simulink model "FilterTest3"  (R2013a)
settings: Solver=FixedStepDiscrete  StartTime=0.0  StopTime=30  RelTol=1e-3
values from neighbouring files (symbols this model uses):
  Ts = 1/100    (= 0.01)    [DataAnalysis.m]
undefined symbols (not defined in the file): a1_1, a1_2, a2_1, a2_2, b0_1, b0_2, b1_1, b1_2, b2_1, b2_2, N, p0_1, p0_2
settings Model: Creator=jban039  LastModifiedBy=jban039

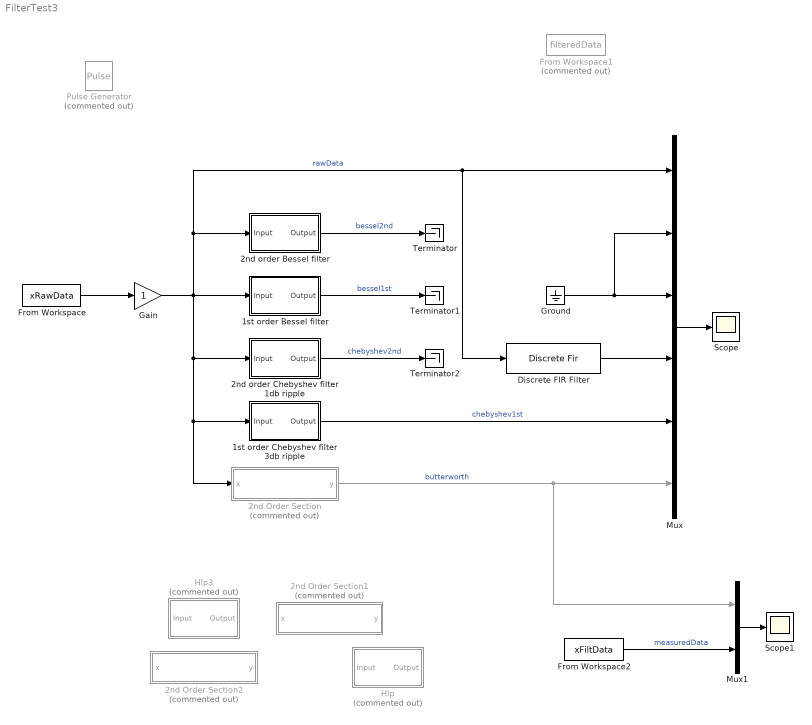
== system FilterTest3 ==
  1st order Bessel filter : Subsystem  Tag=FilterWizardSubSystem
      settings: ErrorFcn=dspFilterRealizedInBasicElemsAlgLoopErrFcnCallback
  1st order Chebyshev filter 3db ripple : Subsystem  Tag=FilterWizardSubSystem
      settings: ErrorFcn=dspFilterRealizedInBasicElemsAlgLoopErrFcnCallback
  2nd Order Section : Subsystem  Tag=FilterWizardSubSystem  Commented=on  mask{Gainp0=141464, Gaina1=-2397004, Gaina2=865708, Gainb0=1, Gainb1=2, Gainb2=1, scalingFactor=21}
      mask prompts: Gainp0 "p_0:"; Gaina1 "a_1:"; Gaina2 "a_2:"; Gainb0 "b_0"; Gainb1 "b_1"; Gainb2 "b_2"
      settings: ErrorFcn=dspFilterRealizedInBasicElemsAlgLoopErrFcnCallback
      mask TypeOptions Gainp0: p0/Gain
      mask TypeOptions Gaina1: a1/Gain
      mask TypeOptions Gaina2: a2/Gain
      mask TypeOptions Gainb0: b0/Gain
      mask TypeOptions Gainb1: b1/Gain
      mask TypeOptions Gainb2: b2/Gain
      mask TypeOptions scalingFactor: scalingFactor/Value
      mask Display:
      | disp('2^{nd} Order Section','interpreter','tex')
      | port_label('input', 1, 'x')
      | port_label('output', 1, 'y')
  2nd Order Section1 : Subsystem  Tag=FilterWizardSubSystem  Commented=on  mask{Gainp0=p0_2, Gaina1=a1_2, Gaina2=a2_2, Gainb0=b0_2, Gainb1=b1_2, Gainb2=b2_2, scalingFactor=N}
      mask prompts: Gainp0 "p_0:"; Gaina1 "a_1:"; Gaina2 "a_2:"; Gainb0 "b_0"; Gainb1 "b_1"; Gainb2 "b_2"
      settings: ErrorFcn=dspFilterRealizedInBasicElemsAlgLoopErrFcnCallback
      mask TypeOptions Gainp0: p0/Gain
      mask TypeOptions Gaina1: a1/Gain
      mask TypeOptions Gaina2: a2/Gain
      mask TypeOptions Gainb0: b0/Gain
      mask TypeOptions Gainb1: b1/Gain
      mask TypeOptions Gainb2: b2/Gain
      mask TypeOptions scalingFactor: scalingFactor/Value
      mask Display:
      | disp('2^{nd} Order Section','interpreter','tex')
      | port_label('input', 1, 'x')
      | port_label('output', 1, 'y')
  2nd Order Section2 : Subsystem  Tag=FilterWizardSubSystem  Commented=on  mask{Gainp0=p0_1, Gaina1=a1_1, Gaina2=a2_1, Gainb0=b0_1, Gainb1=b1_1, Gainb2=b2_1, scalingFactor=N}
      mask prompts: Gainp0 "p_0:"; Gaina1 "a_1:"; Gaina2 "a_2:"; Gainb0 "b_0"; Gainb1 "b_1"; Gainb2 "b_2"
      settings: ErrorFcn=dspFilterRealizedInBasicElemsAlgLoopErrFcnCallback
      mask TypeOptions Gainp0: p0/Gain
      mask TypeOptions Gaina1: a1/Gain
      mask TypeOptions Gaina2: a2/Gain
      mask TypeOptions Gainb0: b0/Gain
      mask TypeOptions Gainb1: b1/Gain
      mask TypeOptions Gainb2: b2/Gain
      mask TypeOptions scalingFactor: scalingFactor/Value
      mask Display:
      | disp('2^{nd} Order Section','interpreter','tex')
      | port_label('input', 1, 'x')
      | port_label('output', 1, 'y')
  2nd order Bessel filter : Subsystem  Tag=FilterWizardSubSystem
      settings: ErrorFcn=dspFilterRealizedInBasicElemsAlgLoopErrFcnCallback
  2nd order Chebyshev filter 1db ripple : Subsystem  Tag=FilterWizardSubSystem
      settings: ErrorFcn=dspFilterRealizedInBasicElemsAlgLoopErrFcnCallback
  Discrete FIR Filter : DiscreteFir  Coefficients=ones(1,16)./16
  From Workspace : FromWorkspace  VariableName=xRawData  SampleTime=0.01  Interpolate=off  OutputAfterFinalValue=Holding final value
  From Workspace1 : FromWorkspace  Commented=on  VariableName=filteredData  SampleTime=0.01  Interpolate=off  OutputAfterFinalValue=Holding final value
  From Workspace2 : FromWorkspace  VariableName=xFiltData  SampleTime=0.01  Interpolate=off  OutputAfterFinalValue=Holding final value
  Gain : Gain
  Ground : Ground
  Hlp : Subsystem  Tag=FilterWizardSubSystem  Commented=on
      settings: ErrorFcn=dspFilterRealizedInBasicElemsAlgLoopErrFcnCallback
  Hlp3 : Subsystem  Tag=FilterWizardSubSystem  Commented=on
      settings: ErrorFcn=dspFilterRealizedInBasicElemsAlgLoopErrFcnCallback
  Mux : Mux  Inputs=6
  Mux1 : Mux  Inputs=2
  Pulse Generator : DiscretePulseGenerator  Commented=on  PulseType=Time based  Period=0.4  PulseWidth=50
  Scope : Scope
      settings: ShowLegends=on  TimeRange=30  YMin=-100  YMax=300
  Scope1 : Scope
      settings: ShowLegends=on  TimeRange=1  YMin=0  YMax=300
  Terminator : Terminator
  Terminator1 : Terminator
  Terminator2 : Terminator
  wires:
  From Workspace/1 -> Gain/1
  Gain/1 -> 2nd order Bessel filter/1(Input), Discrete FIR Filter/1, Mux/1, 2nd Order Section/1(x), 1st order Chebyshev filter 3db ripple/1(Input), 2nd order Chebyshev filter 1db ripple/1(Input), 1st order Bessel filter/1(Input)  "rawData"
  2nd order Bessel filter/1(Output) -> Terminator/1  "bessel2nd"
  Mux/1 -> Scope/1
  1st order Bessel filter/1(Output) -> Terminator1/1  "bessel1st"
  2nd order Chebyshev filter 1db ripple/1(Output) -> Terminator2/1  "chebyshev2nd"
  1st order Chebyshev filter 3db ripple/1(Output) -> Mux/5  "chebyshev1st"
  2nd Order Section/1(y) -> Mux1/1, Mux/6  "butterworth"
  From Workspace2/1 -> Mux1/2  "measuredData"
  Mux1/1 -> Scope1/1
  Ground/1 -> Mux/3, Mux/2
  Discrete FIR Filter/1 -> Mux/4

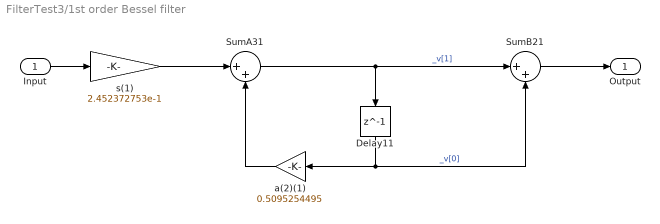
== system FilterTest3/1st order Bessel filter ==
  Input : Inport
  Delay11 : Delay  DelayLength=1  InitialCondition=0  SampleTime=Ts
  SumA31 : Sum  Inputs=|++  RndMeth=Nearest  SaturateOnIntegerOverflow=on  OutDataTypeStr=Inherit: Same as first input
  SumB21 : Sum  Inputs=|++  RndMeth=Nearest  SaturateOnIntegerOverflow=on  OutDataTypeStr=Inherit: Same as first input
  a(2)(1) : Gain  Gain=0.5095254495  ParamDataTypeStr=double  RndMeth=Nearest  SaturateOnIntegerOverflow=on  OutDataTypeStr=Inherit: Same as input
  s(1) : Gain  Gain=2.452372753e-1  ParamDataTypeStr=double  RndMeth=Nearest  SaturateOnIntegerOverflow=on  OutDataTypeStr=Inherit: Same as input
  Output : Outport
  wires:
  SumB21/1 -> Output/1
  s(1)/1 -> SumA31/1
  Delay11/1 -> SumB21/2, a(2)(1)/1  "_v[0]"
  a(2)(1)/1 -> SumA31/2
  SumA31/1 -> Delay11/1, SumB21/1  "_v[1]"
  Input/1 -> s(1)/1

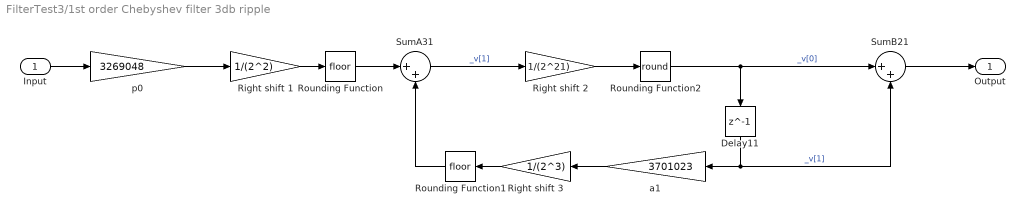
== system FilterTest3/1st order Chebyshev filter 3db ripple ==
  Input : Inport
  Delay11 : Delay  DelayLength=1  InitialCondition=0  SampleTime=Ts
  Right shift 1 : Gain  Gain=1/(2^2)  ParamDataTypeStr=double  RndMeth=Nearest  SaturateOnIntegerOverflow=on  OutDataTypeStr=Inherit: Same as input
  Right shift 2 : Gain  Gain=1/(2^21)  ParamDataTypeStr=double  RndMeth=Nearest  SaturateOnIntegerOverflow=on  OutDataTypeStr=Inherit: Same as input
  Right shift 3 : Gain  Gain=1/(2^3)  ParamDataTypeStr=double  RndMeth=Nearest  SaturateOnIntegerOverflow=on  OutDataTypeStr=Inherit: Same as input
  Rounding Function : Rounding
  Rounding Function1 : Rounding
  Rounding Function2 : Rounding  Operator=round
  SumA31 : Sum  Inputs=|++  RndMeth=Nearest  SaturateOnIntegerOverflow=on  OutDataTypeStr=Inherit: Same as first input
  SumB21 : Sum  Inputs=|++  RndMeth=Nearest  SaturateOnIntegerOverflow=on  OutDataTypeStr=Inherit: Same as first input
  a1 : Gain  Gain=3701023  ParamDataTypeStr=double  RndMeth=Nearest  SaturateOnIntegerOverflow=on  OutDataTypeStr=Inherit: Same as input
  p0 : Gain  Gain=3269048  ParamDataTypeStr=double  RndMeth=Nearest  SaturateOnIntegerOverflow=on  OutDataTypeStr=Inherit: Same as input
  Output : Outport
  wires:
  Input/1 -> p0/1
  SumA31/1 -> Right shift 2/1  "_v[1]"
  a1/1 -> Right shift 3/1
  Delay11/1 -> a1/1, SumB21/2  "_v[1]"
  p0/1 -> Right shift 1/1
  SumB21/1 -> Output/1
  Right shift 1/1 -> Rounding Function/1
  Rounding Function/1 -> SumA31/1
  Rounding Function1/1 -> SumA31/2
  Right shift 3/1 -> Rounding Function1/1
  Right shift 2/1 -> Rounding Function2/1
  Rounding Function2/1 -> SumB21/1, Delay11/1  "_v[0]"

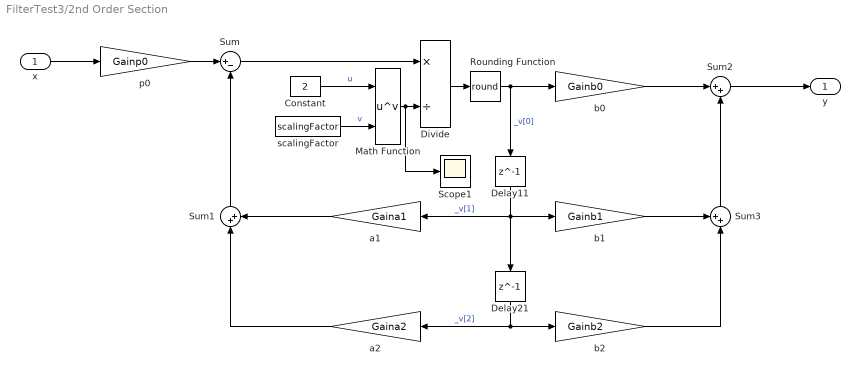
== system FilterTest3/2nd Order Section ==
  x : Inport
  Constant : Constant  Value=2
  Delay11 : Delay  DelayLength=1  InitialCondition=0  SampleTime=Ts
  Delay21 : Delay  DelayLength=1  InitialCondition=0  SampleTime=Ts
  Divide : Product  Inputs=*/
  Math Function : Math  Operator=pow  SaturateOnIntegerOverflow=on
  Rounding Function : Rounding  Operator=round
  Scope1 : Scope
      settings: ShowLegends=on  TimeRange=60  YMin=-100  YMax=300  SaveName=ScopeData2
  Sum : Sum  Inputs=|+-
  Sum1 : Sum  Inputs=|++
  Sum2 : Sum  Inputs=|++
  Sum3 : Sum  Inputs=++|
  a1 : Gain  Gain=Gaina1  ParamDataTypeStr=double  RndMeth=Nearest  SaturateOnIntegerOverflow=on  OutDataTypeStr=Inherit: Same as input
  a2 : Gain  Gain=Gaina2  ParamDataTypeStr=double  RndMeth=Nearest  SaturateOnIntegerOverflow=on  OutDataTypeStr=Inherit: Same as input
  b0 : Gain  Gain=Gainb0  ParamDataTypeStr=double  RndMeth=Nearest  SaturateOnIntegerOverflow=on  OutDataTypeStr=Inherit: Same as input
  b1 : Gain  Gain=Gainb1  ParamDataTypeStr=double  RndMeth=Nearest  SaturateOnIntegerOverflow=on  OutDataTypeStr=Inherit: Same as input
  b2 : Gain  Gain=Gainb2  ParamDataTypeStr=double  RndMeth=Nearest  SaturateOnIntegerOverflow=on  OutDataTypeStr=Inherit: Same as input
  p0 : Gain  Gain=Gainp0  ParamDataTypeStr=double  RndMeth=Nearest  SaturateOnIntegerOverflow=on  OutDataTypeStr=Inherit: Same as input
  scalingFactor : Constant  Value=scalingFactor
  y : Outport
  wires:
  p0/1 -> Sum/1
  Delay21/1 -> b2/1, a2/1  "_v[2]"
  a2/1 -> Sum1/1
  b1/1 -> Sum3/1
  Delay11/1 -> b1/1, a1/1, Delay21/1  "_v[1]"
  a1/1 -> Sum1/2
  Rounding Function/1 -> b0/1, Delay11/1  "_v[0]"
  x/1 -> p0/1
  Sum1/1 -> Sum/2
  Sum3/1 -> Sum2/2
  b0/1 -> Sum2/1
  b2/1 -> Sum3/2
  Sum2/1 -> y/1
  Sum/1 -> Divide/1
  Divide/1 -> Rounding Function/1
  Constant/1 -> Math Function/1  "u"
  scalingFactor/1 -> Math Function/2  "v"
  Math Function/1 -> Scope1/1, Divide/2

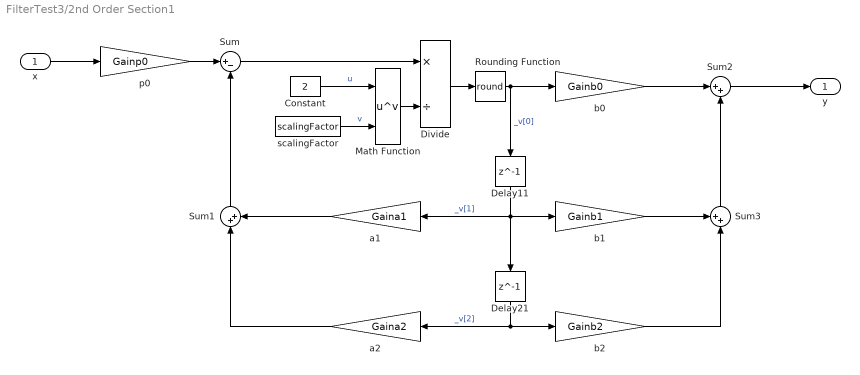
== system FilterTest3/2nd Order Section1 ==
  x : Inport
  Constant : Constant  Value=2
  Delay11 : Delay  DelayLength=1  InitialCondition=0  SampleTime=Ts
  Delay21 : Delay  DelayLength=1  InitialCondition=0  SampleTime=Ts
  Divide : Product  Inputs=*/
  Math Function : Math  Operator=pow  SaturateOnIntegerOverflow=on
  Rounding Function : Rounding  Operator=round
  Sum : Sum  Inputs=|+-
  Sum1 : Sum  Inputs=|++
  Sum2 : Sum  Inputs=|++
  Sum3 : Sum  Inputs=++|
  a1 : Gain  Gain=Gaina1  ParamDataTypeStr=double  RndMeth=Nearest  SaturateOnIntegerOverflow=on  OutDataTypeStr=Inherit: Same as input
  a2 : Gain  Gain=Gaina2  ParamDataTypeStr=double  RndMeth=Nearest  SaturateOnIntegerOverflow=on  OutDataTypeStr=Inherit: Same as input
  b0 : Gain  Gain=Gainb0  ParamDataTypeStr=double  RndMeth=Nearest  SaturateOnIntegerOverflow=on  OutDataTypeStr=Inherit: Same as input
  b1 : Gain  Gain=Gainb1  ParamDataTypeStr=double  RndMeth=Nearest  SaturateOnIntegerOverflow=on  OutDataTypeStr=Inherit: Same as input
  b2 : Gain  Gain=Gainb2  ParamDataTypeStr=double  RndMeth=Nearest  SaturateOnIntegerOverflow=on  OutDataTypeStr=Inherit: Same as input
  p0 : Gain  Gain=Gainp0  ParamDataTypeStr=double  RndMeth=Nearest  SaturateOnIntegerOverflow=on  OutDataTypeStr=Inherit: Same as input
  scalingFactor : Constant  Value=scalingFactor
  y : Outport
  wires:
  Math Function/1 -> Divide/2
  scalingFactor/1 -> Math Function/2  "v"
  Constant/1 -> Math Function/1  "u"
  Divide/1 -> Rounding Function/1
  Sum/1 -> Divide/1
  Sum2/1 -> y/1
  b2/1 -> Sum3/2
  b0/1 -> Sum2/1
  Sum3/1 -> Sum2/2
  Sum1/1 -> Sum/2
  x/1 -> p0/1
  Rounding Function/1 -> Delay11/1, b0/1  "_v[0]"
  a1/1 -> Sum1/2
  Delay11/1 -> Delay21/1, a1/1, b1/1  "_v[1]"
  b1/1 -> Sum3/1
  a2/1 -> Sum1/1
  Delay21/1 -> a2/1, b2/1  "_v[2]"
  p0/1 -> Sum/1

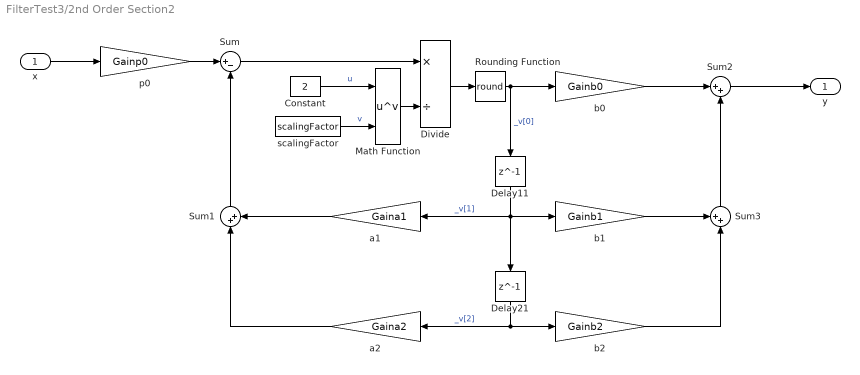
== system FilterTest3/2nd Order Section2 ==
  x : Inport
  Constant : Constant  Value=2
  Delay11 : Delay  DelayLength=1  InitialCondition=0  SampleTime=Ts
  Delay21 : Delay  DelayLength=1  InitialCondition=0  SampleTime=Ts
  Divide : Product  Inputs=*/
  Math Function : Math  Operator=pow  SaturateOnIntegerOverflow=on
  Rounding Function : Rounding  Operator=round
  Sum : Sum  Inputs=|+-
  Sum1 : Sum  Inputs=|++
  Sum2 : Sum  Inputs=|++
  Sum3 : Sum  Inputs=++|
  a1 : Gain  Gain=Gaina1  ParamDataTypeStr=double  RndMeth=Nearest  SaturateOnIntegerOverflow=on  OutDataTypeStr=Inherit: Same as input
  a2 : Gain  Gain=Gaina2  ParamDataTypeStr=double  RndMeth=Nearest  SaturateOnIntegerOverflow=on  OutDataTypeStr=Inherit: Same as input
  b0 : Gain  Gain=Gainb0  ParamDataTypeStr=double  RndMeth=Nearest  SaturateOnIntegerOverflow=on  OutDataTypeStr=Inherit: Same as input
  b1 : Gain  Gain=Gainb1  ParamDataTypeStr=double  RndMeth=Nearest  SaturateOnIntegerOverflow=on  OutDataTypeStr=Inherit: Same as input
  b2 : Gain  Gain=Gainb2  ParamDataTypeStr=double  RndMeth=Nearest  SaturateOnIntegerOverflow=on  OutDataTypeStr=Inherit: Same as input
  p0 : Gain  Gain=Gainp0  ParamDataTypeStr=double  RndMeth=Nearest  SaturateOnIntegerOverflow=on  OutDataTypeStr=Inherit: Same as input
  scalingFactor : Constant  Value=scalingFactor
  y : Outport
  wires:
  Math Function/1 -> Divide/2
  scalingFactor/1 -> Math Function/2  "v"
  Constant/1 -> Math Function/1  "u"
  Divide/1 -> Rounding Function/1
  Sum/1 -> Divide/1
  Sum2/1 -> y/1
  b2/1 -> Sum3/2
  b0/1 -> Sum2/1
  Sum3/1 -> Sum2/2
  Sum1/1 -> Sum/2
  x/1 -> p0/1
  Rounding Function/1 -> Delay11/1, b0/1  "_v[0]"
  a1/1 -> Sum1/2
  Delay11/1 -> Delay21/1, a1/1, b1/1  "_v[1]"
  b1/1 -> Sum3/1
  a2/1 -> Sum1/1
  Delay21/1 -> a2/1, b2/1  "_v[2]"
  p0/1 -> Sum/1

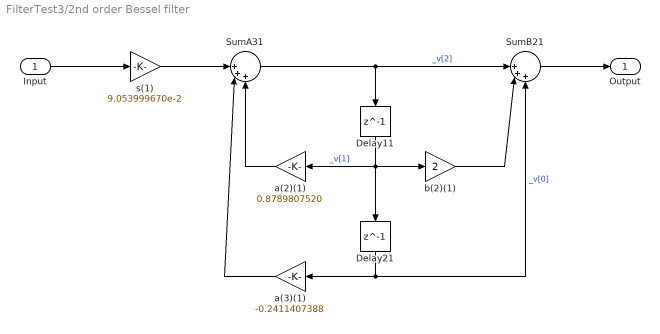
== system FilterTest3/2nd order Bessel filter ==
  Input : Inport
  Delay11 : Delay  DelayLength=1  InitialCondition=0  SampleTime=Ts
  Delay21 : Delay  DelayLength=1  InitialCondition=0  SampleTime=Ts
  SumA31 : Sum  Inputs=||+++  RndMeth=Nearest  SaturateOnIntegerOverflow=on  OutDataTypeStr=Inherit: Same as first input
  SumB21 : Sum  Inputs=||+++  RndMeth=Nearest  SaturateOnIntegerOverflow=on  OutDataTypeStr=Inherit: Same as first input
  a(2)(1) : Gain  Gain=0.8789807520  ParamDataTypeStr=double  RndMeth=Nearest  SaturateOnIntegerOverflow=on  OutDataTypeStr=Inherit: Same as input
  a(3)(1) : Gain  Gain=-0.2411407388  ParamDataTypeStr=double  RndMeth=Nearest  SaturateOnIntegerOverflow=on  OutDataTypeStr=Inherit: Same as input
  b(2)(1) : Gain  Gain=2  ParamDataTypeStr=double  RndMeth=Nearest  SaturateOnIntegerOverflow=on  OutDataTypeStr=Inherit: Same as input
  s(1) : Gain  Gain=9.053999670e-2  ParamDataTypeStr=double  RndMeth=Nearest  SaturateOnIntegerOverflow=on  OutDataTypeStr=Inherit: Same as input
  Output : Outport
  wires:
  Input/1 -> s(1)/1
  SumA31/1 -> SumB21/1, Delay11/1  "_v[2]"
  a(2)(1)/1 -> SumA31/3
  Delay11/1 -> Delay21/1, a(2)(1)/1, b(2)(1)/1  "_v[1]"
  b(2)(1)/1 -> SumB21/2
  a(3)(1)/1 -> SumA31/2
  Delay21/1 -> SumB21/3, a(3)(1)/1  "_v[0]"
  s(1)/1 -> SumA31/1
  SumB21/1 -> Output/1

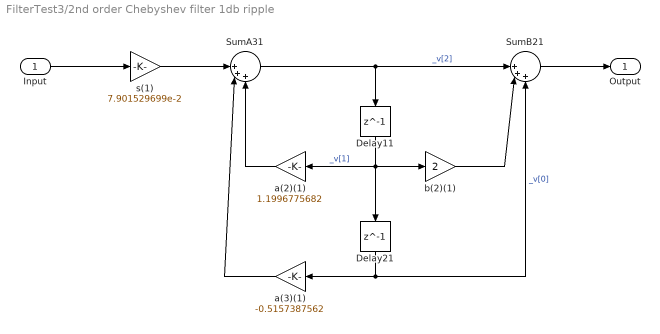
== system FilterTest3/2nd order Chebyshev filter 1db ripple ==
  Input : Inport
  Delay11 : Delay  DelayLength=1  InitialCondition=0  SampleTime=Ts
  Delay21 : Delay  DelayLength=1  InitialCondition=0  SampleTime=Ts
  SumA31 : Sum  Inputs=||+++  RndMeth=Nearest  SaturateOnIntegerOverflow=on  OutDataTypeStr=Inherit: Same as first input
  SumB21 : Sum  Inputs=||+++  RndMeth=Nearest  SaturateOnIntegerOverflow=on  OutDataTypeStr=Inherit: Same as first input
  a(2)(1) : Gain  Gain=1.1996775682  ParamDataTypeStr=double  RndMeth=Nearest  SaturateOnIntegerOverflow=on  OutDataTypeStr=Inherit: Same as input
  a(3)(1) : Gain  Gain=-0.5157387562  ParamDataTypeStr=double  RndMeth=Nearest  SaturateOnIntegerOverflow=on  OutDataTypeStr=Inherit: Same as input
  b(2)(1) : Gain  Gain=2  ParamDataTypeStr=double  RndMeth=Nearest  SaturateOnIntegerOverflow=on  OutDataTypeStr=Inherit: Same as input
  s(1) : Gain  Gain=7.901529699e-2  ParamDataTypeStr=double  RndMeth=Nearest  SaturateOnIntegerOverflow=on  OutDataTypeStr=Inherit: Same as input
  Output : Outport
  wires:
  SumB21/1 -> Output/1
  s(1)/1 -> SumA31/1
  Delay21/1 -> a(3)(1)/1, SumB21/3  "_v[0]"
  a(3)(1)/1 -> SumA31/2
  b(2)(1)/1 -> SumB21/2
  Delay11/1 -> b(2)(1)/1, a(2)(1)/1, Delay21/1  "_v[1]"
  a(2)(1)/1 -> SumA31/3
  SumA31/1 -> Delay11/1, SumB21/1  "_v[2]"
  Input/1 -> s(1)/1

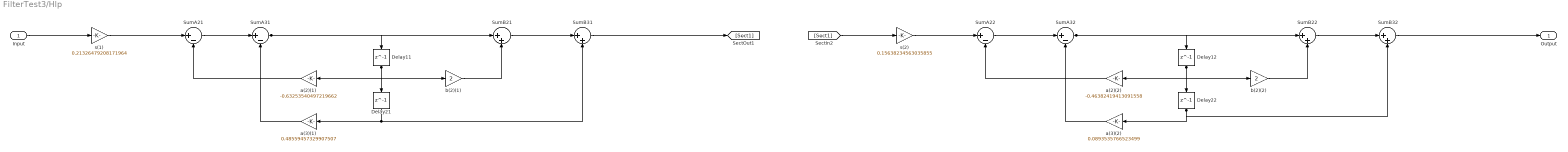
== system FilterTest3/Hlp ==
  Input : Inport
  Delay{11..12,21..22} (4 alike) : Delay  DelayLength=1  InitialCondition=0
  SumA{21..22,31..32} (4 alike) : Sum  Inputs=|+-  RndMeth=Nearest  SaturateOnIntegerOverflow=on  OutDataTypeStr=Inherit: Same as first input
  SumB{21..22,31..32} (4 alike) : Sum  Inputs=|++  RndMeth=Nearest  SaturateOnIntegerOverflow=on  OutDataTypeStr=Inherit: Same as first input
  a(2)(1) : Gain  Gain=-0.63253540497219662  ParamDataTypeStr=double  RndMeth=Nearest  SaturateOnIntegerOverflow=on  OutDataTypeStr=Inherit: Same as input
  a(2)(2) : Gain  Gain=-0.46382419413091558  ParamDataTypeStr=double  RndMeth=Nearest  SaturateOnIntegerOverflow=on  OutDataTypeStr=Inherit: Same as input
  a(3)(1) : Gain  Gain=0.48559457329907507  ParamDataTypeStr=double  RndMeth=Nearest  SaturateOnIntegerOverflow=on  OutDataTypeStr=Inherit: Same as input
  a(3)(2) : Gain  Gain=0.0893535766523499  ParamDataTypeStr=double  RndMeth=Nearest  SaturateOnIntegerOverflow=on  OutDataTypeStr=Inherit: Same as input
  b(2)(1) : Gain  Gain=2  ParamDataTypeStr=double  RndMeth=Nearest  SaturateOnIntegerOverflow=on  OutDataTypeStr=Inherit: Same as input
  b(2)(2) : Gain  Gain=2  ParamDataTypeStr=double  RndMeth=Nearest  SaturateOnIntegerOverflow=on  OutDataTypeStr=Inherit: Same as input
  s(1) : Gain  Gain=0.21326479208171964  ParamDataTypeStr=double  RndMeth=Nearest  SaturateOnIntegerOverflow=on  OutDataTypeStr=Inherit: Same as input
  s(2) : Gain  Gain=0.15638234563035855  ParamDataTypeStr=double  RndMeth=Nearest  SaturateOnIntegerOverflow=on  OutDataTypeStr=Inherit: Same as input
  Output : Outport
  wires:
  Input/1 -> s(1)/1
  s(1)/1 -> SumA21/1
  SumA21/1 -> SumA31/1
  SumA31/1 -> SumB21/1, Delay11/1
  SumB21/1 -> SumB31/1
  SumB31/1 -> [Sect1]
  a(2)(1)/1 -> SumA21/2
  Delay11/1 -> a(2)(1)/1, b(2)(1)/1, Delay21/1
  b(2)(1)/1 -> SumB21/2
  a(3)(1)/1 -> SumA31/2
  Delay21/1 -> a(3)(1)/1, SumB31/2
  [Sect1] -> s(2)/1
  s(2)/1 -> SumA22/1
  SumA22/1 -> SumA32/1
  SumA32/1 -> SumB22/1, Delay12/1
  SumB22/1 -> SumB32/1
  SumB32/1 -> Output/1
  a(2)(2)/1 -> SumA22/2
  Delay12/1 -> a(2)(2)/1, b(2)(2)/1, Delay22/1
  b(2)(2)/1 -> SumB22/2
  a(3)(2)/1 -> SumA32/2
  Delay22/1 -> a(3)(2)/1, SumB32/2

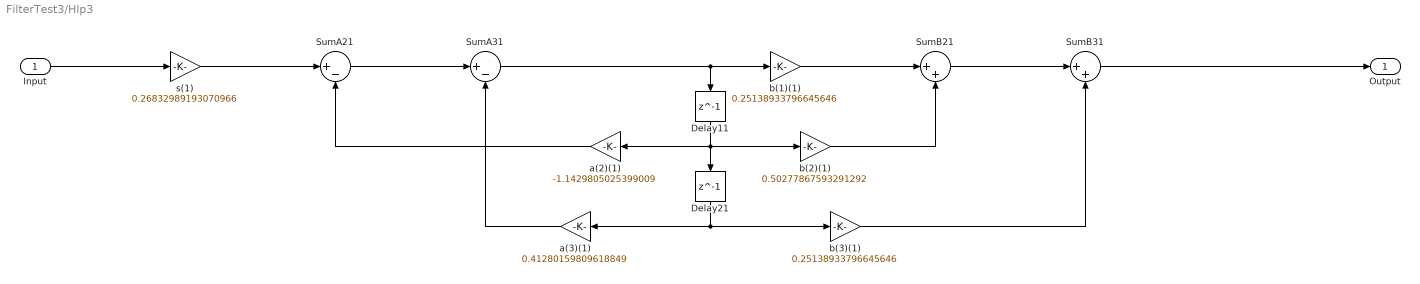
== system FilterTest3/Hlp3 ==
  Input : Inport
  Delay11 : Delay  DelayLength=1  InitialCondition=0
  Delay21 : Delay  DelayLength=1  InitialCondition=0
  SumA21 : Sum  Inputs=|+-  RndMeth=Nearest  SaturateOnIntegerOverflow=on  OutDataTypeStr=Inherit: Same as first input
  SumA31 : Sum  Inputs=|+-  RndMeth=Nearest  SaturateOnIntegerOverflow=on  OutDataTypeStr=Inherit: Same as first input
  SumB21 : Sum  Inputs=|++  RndMeth=Nearest  SaturateOnIntegerOverflow=on  OutDataTypeStr=Inherit: Same as first input
  SumB31 : Sum  Inputs=|++  RndMeth=Nearest  SaturateOnIntegerOverflow=on  OutDataTypeStr=Inherit: Same as first input
  a(2)(1) : Gain  Gain=-1.1429805025399009  ParamDataTypeStr=double  RndMeth=Nearest  SaturateOnIntegerOverflow=on  OutDataTypeStr=Inherit: Same as input
  a(3)(1) : Gain  Gain=0.41280159809618849  ParamDataTypeStr=double  RndMeth=Nearest  SaturateOnIntegerOverflow=on  OutDataTypeStr=Inherit: Same as input
  b(1)(1) : Gain  Gain=0.25138933796645646  ParamDataTypeStr=double  RndMeth=Nearest  SaturateOnIntegerOverflow=on  OutDataTypeStr=Inherit: Same as input
  b(2)(1) : Gain  Gain=0.50277867593291292  ParamDataTypeStr=double  RndMeth=Nearest  SaturateOnIntegerOverflow=on  OutDataTypeStr=Inherit: Same as input
  b(3)(1) : Gain  Gain=0.25138933796645646  ParamDataTypeStr=double  RndMeth=Nearest  SaturateOnIntegerOverflow=on  OutDataTypeStr=Inherit: Same as input
  s(1) : Gain  Gain=0.26832989193070966  ParamDataTypeStr=double  RndMeth=Nearest  SaturateOnIntegerOverflow=on  OutDataTypeStr=Inherit: Same as input
  Output : Outport
  wires:
  Input/1 -> s(1)/1
  s(1)/1 -> SumA21/1
  SumA21/1 -> SumA31/1
  SumA31/1 -> b(1)(1)/1, Delay11/1
  b(1)(1)/1 -> SumB21/1
  SumB21/1 -> SumB31/1
  SumB31/1 -> Output/1
  a(2)(1)/1 -> SumA21/2
  Delay11/1 -> a(2)(1)/1, b(2)(1)/1, Delay21/1
  b(2)(1)/1 -> SumB21/2
  a(3)(1)/1 -> SumA31/2
  Delay21/1 -> a(3)(1)/1, b(3)(1)/1
  b(3)(1)/1 -> SumB31/2
